simulink model "Switching_Preisach"  (R2017b)
settings: Solver=FixedStepAuto  StartTime=0.0  StopTime=simTotalTime  FixedStep=0.05  MaxStep=0.1  MinStep=0.01  RelTol=1e-3
undefined symbols (not defined in the file): GA, GB, GC, GD, gridArea, gridDen, gridLength, Gx0, hysteronMax, hysteronMin, initialRelays, inputFactor, inputMax, inputMin, offset, outputFactor, outputMax, outputMin, weightFunc, xyGrid
libraries: simulink x2
settings Model: Creator=Marco  LastModifiedBy=M. Vasquez Beltran

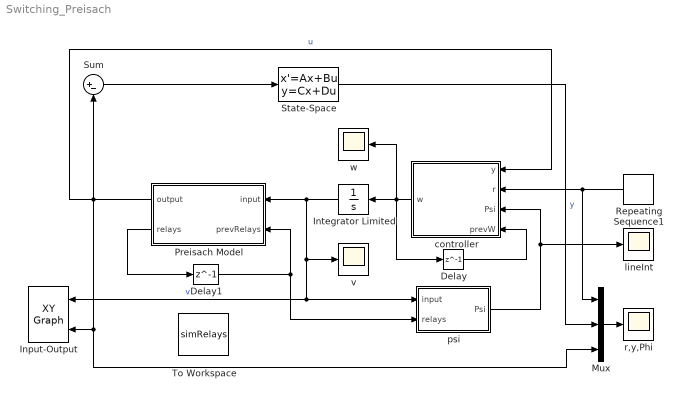
== system Switching_Preisach ==
  Delay : Delay  DelayLength=1
  Delay1 : Delay  DelayLength=1  InitialCondition=initialRelays
  Input-Output : simulink/Sinks/XY Graph  xmin=inputMin*inputFactor  xmax=inputMax*inputFactor  ymin=outputMin*outputFactor  ymax=outputMax*outputFactor  st=-1
  Integrator Limited : Integrator  InitialCondition=0.75  UpperSaturationLimit=inputMax*0.99  LowerSaturationLimit=inputMin*0.99
  Mux : Mux  Inputs=3
  Preisach Model : MATLAB Function  TreatAsAtomicUnit=on
  Repeating Sequence1 : simulink/Sources/Repeating Sequence  rep_seq_t=sequenceTime  rep_seq_y=sequenceVal
  State-Space : StateSpace  A=GA  B=GB  C=GC  D=GD  InitialCondition=Gx0
  Sum : Sum  Inputs=|+-
  To Workspace : ToWorkspace  VariableName=simRelays  SampleTime=-1
  controller : MATLAB Function  TreatAsAtomicUnit=on
  lineInt : Scope
  psi : MATLAB Function  TreatAsAtomicUnit=on
  r,y,Phi : Scope
  v : Scope
  w : Scope
  wires:
  Preisach Model/2(relays) -> Delay1/1
  Delay1/1 -> Preisach Model/2(prevRelays), psi/2(relays)
  Sum/1 -> State-Space/1
  Preisach Model/1(output) -> controller/1(y), Sum/2, Input-Output/2, Mux/3  "u"
  State-Space/1 -> Mux/2  "y"
  Integrator Limited/1 -> psi/1(input), Input-Output/1, v/1, Preisach Model/1(input)  "v"
  Repeating Sequence1/1 -> Mux/1, controller/2(r)
  controller/1(w) -> Delay/1, Integrator Limited/1, w/1
  Mux/1 -> r,y,Phi/1
  Delay/1 -> controller/4(prevW)
  psi/1(Psi) -> lineInt/1, controller/3(Psi)

== matlab function Switching_Preisach/Preisach Model ==
  data: input input; prevRelays input; output output; weightFunc parameter; relays output; offset parameter; hysteronMin parameter; hysteronMax parameter; gridDen parameter; xyGrid parameter; gridLength parameter; gridArea parameter
function [output, relays] = fcn(input, prevRelays, ...
    weightFunc, offset, hysteronMin, hysteronMax, gridDen, xyGrid, gridLength, gridArea)

%     output = offset;
%     relays = prevRelays;
%     for i=1:gridDen
%         ii = gridDen-i+1; %index inversion for rows
%         for j=1:i
%             if( input >= xyGrid(i) && relays(ii,j) ~= hysteronMax )
%                 relays(ii,j) = hysteronMax;
%             elseif( input <= xyGrid(j) && relays(ii,j) ~= hysteronMin )
%                 relays(ii,j) = hysteronMin;
%             end
%             output = output + relays(ii,j)*weightFunc(ii,j)*gridArea;
%         end
%     end



%     relays = prevRelays;
%     for row=1:gridDen+1
%         if( row == gridDen+1 || input <= xyGrid(row) )
%             row = row-1;
%             irow = gridDen-row+1;
%             relays(irow:end, 1:row) = hysteronMax*fliplr(triu(ones(row, row)));
%             break;
%         end
%     end
%     for col=gridDen:-1:0
%         if( col == 0 || input >= xyGrid(col) )
%             col = col+1;
%             irow = gridDen-col+1;
%             relays(1:irow, col:end) = hysteronMin*fliplr(triu(ones(irow, irow)));
%             break;
%         end
%     end
%     output = sum(sum(relays(:,:).*weightFunc(:,:)))*gridArea + offset;



    relays = prevRelays;
    if( xyGrid(end) <= input )
        relays(:,:) = hysteronMax*fliplr(triu(ones(gridDen, gridDen)));
    elseif( input < xyGrid(1) )
        relays(:,:) = hysteronMin*fliplr(triu(ones(gridDen, gridDen)));
    else
        idx0 = 1;
        while( idx0 <= gridDen-1 )
            if( xyGrid(idx0) <= input && input < xyGrid(idx0+1) )
                col = idx0;
                row = gridDen-idx0+1;

                relays(row:end, 1:col) = hysteronMax*fliplr(triu(ones(col, col)));
                relays(1:row-1, col+1:end) = hysteronMin*fliplr(triu(ones(row-1, row-1)));
                break;
            end
            idx0 = idx0 + 1;
        end
    end
    output = sum(sum(relays(:,:).*weightFunc(:,:)))*gridArea + offset;

== matlab function Switching_Preisach/psi ==
  data: input input; relays input; weightFunc parameter; hysteronMin parameter; hysteronMax parameter; offset parameter; gridDen parameter; Psi output; xyGrid parameter; gridLength parameter
function Psi = fcn(input, relays,...
     weightFunc, hysteronMin, hysteronMax, offset, gridDen, xyGrid, gridLength)

Psi = [0; 0];
if( xyGrid(end) <= input )
    return;
elseif( input < xyGrid(1) )
    return;
else
    idx0 = 1;
    while( idx0 <= gridDen-1 )
        if( xyGrid(idx0) <= input && input < xyGrid(idx0+1) )
            col = idx0;
            row = gridDen-idx0+1;
            
            for var=col:-1:1
                if( relays(row-1,var)==hysteronMin )
                    Psi(1) = Psi(1) + gridLength*weightFunc(row-1,var);
                end
            end
            
            for var=row:-1:1
                if( relays(var,col)==hysteronMax )
                    Psi(2) = Psi(2) + gridLength*weightFunc(var,col);
                end
            end
            
            break;
        end
        idx0 = idx0 + 1;
    end
end
Psi = 2*Psi;

end

== matlab function Switching_Preisach/controller ==
  data: y input; r input; Psi input; prevW input; w output
function w = fcn(y,r,Psi,prevW)
    
    % Error
    e = r-y;
    
    %%%%%%%%%%%%%%%%%%%%%%%%%%%%%%%%%%%%%%%%%%%%%%%%%%%%%%%%%%%%%%%%%%%%%%%
    % Selecting the last value of nonliearity psi
    %%%%%%%%%%%%%%%%%%%%%%%%%%%%%%%%%%%%%%%%%%%%%%%%%%%%%%%%%%%%%%%%%%%%%%%
    if(sign(prevW)>0)
        prevPsi=Psi(1);
    elseif(sign(prevW)<0)
        prevPsi=Psi(2);
    else
        prevPsi=0;
    end
    %%%%%%%%%%%%%%%%%%%%%%%%%%%%%%%%%%%%%%%%%%%%%%%%%%%%%%%%%%%%%%%%%%%%%%%
    
    %%%%%%%%%%%%%%%%%%%%%%%%%%%%%%%%%%%%%%%%%%%%%%%%%%%%%%%%%%%%%%%%%%%%%%%
    % Control logic
    %%%%%%%%%%%%%%%%%%%%%%%%%%%%%%%%%%%%%%%%%%%%%%%%%%%%%%%%%%%%%%%%%%%%%%%
    if(e==0)
        w=0;
    elseif(sign(prevPsi)==0 || abs(prevPsi)<0.25)
        if(prevW==0)
            w = e;
        else
            w = abs(e)*sign(prevW);
        end
    else
        w = e*sign(prevPsi);
    end
    %%%%%%%%%%%%%%%%%%%%%%%%%%%%%%%%%%%%%%%%%%%%%%%%%%%%%%%%%%%%%%%%%%%%%%%
    
    
%     k = 2;
%     lineIntTh = 0.1;

%     if( abs(Psi(1)) <= lineIntTh && abs(Psi(2)) <= lineIntTh )
%         w = 0;
%     elseif( abs(Psi(1)) >= abs(Psi(2)) )
%         w = k*(r-y)/Psi(1);
%     else
%         w = -k*(r-y)/Psi(2);
%     end
    
%     w = 0;
%     signVec = Psi;
%     signVec(signVec>=0) = 1;
%     signVec(signVec<0) = -1;
%     if( abs(Psi(1)) > abs(Psi(2)) )
%         lambda = signVec(1)*max(abs([Psi(1), lineIntTh]));
%     else
%         lambda = signVec(2)*max(abs([Psi(2), lineIntTh]));
%     end
%     w = k*(r-y)/lambda;

%%%%%%%%%%%%%%%%%%%%%
% Working
%%%%%%%%%%%%%%%%%%%%%
%     w = 0;
%     if( r-y>0 )
%         lambda = max(abs([Psi(1), lineIntTh]));
%     else
%         lambda = max(abs([Psi(2), lineIntTh]));
%     end
%     w = k*(r-y)/lambda;
%%%%%%%%%%%%%%%%%%%%%
    
%     w = 0;
%     e = r-y;
%     if ( e>0 )
%         if ( Psi(1)>0 )
%             w =  abs(e)/max(abs([lineIntTh, Psi(1)]));
%         elseif ( Psi(2)<0 )
%             w = -abs(e)/max(abs([lineIntTh, Psi(2)]));
%         elseif ( Psi(1)<=0 )
%             w = -abs(e)/max(abs([lineIntTh, Psi(2)]));
%         end
%     elseif( e<0 )
%         if ( Psi(2)>0 )
%             w = -abs(e)/max(abs([lineIntTh, Psi(2)]));
%         elseif ( Psi(1)<0 )
%             w =  abs(e)/max(abs([lineIntTh, Psi(1)]));
%         elseif ( Psi(2)<=0 )
%             w = abs(e)/max(abs([lineIntTh, Psi(1)]));
%         end
%     end
    
end
